simulink model "discrete_model"  (R2024b)
settings: Solver=VariableStepAuto  StartTime=0.0  StopTime=10.0  MaxStep=1e-4  RelTol=1e-3
values from neighbouring files (symbols this model uses):
  A = [0,1; 0,-10]    [conti_ss_script.m]    (also in discrete_script.m = [0,1; -3, -60]; error_space_script.m = [0,1; 0,-20]; observer_script.m = [0,1; 0,-20]; pid_script.m)
  B = [0; 120]    [conti_ss_script.m]    (also in discrete_script.m = [0; 1]; error_space_script.m = [0; 60]; observer_script.m = [0; 60]; pid_script.m)
  C = [1, 0]    [conti_ss_script.m]    (also in discrete_script.m = [90, 0]; error_space_script.m = [1,0]; observer_script.m = [1,0]; pid_script.m)
  D = 0    [conti_ss_script.m]    (also in discrete_script.m; error_space_script.m; observer_script.m; pid_script.m)
  GamO = GamOO    [discrete_script.m]
  HO = HOO    [discrete_script.m]
  JO = JOO    [discrete_script.m]
  K = Ke(2:end)    [conti_ss_script.m]    (also in discrete_script.m = Kdd; error_space_script.m = Kz(4:5); observer_script.m)
  Nu = ff(3)    [conti_ss_script.m]    (also in discrete_script.m = Nudd; observer_script.m)
  Nx = ff(1:2)    [conti_ss_script.m]    (also in discrete_script.m = Nxdd; observer_script.m)
  PhiO = PhiOO    [discrete_script.m]
  Ts = 1e-3    (= 0.001)    [discrete_script.m]
settings Model: Creator=pries  LastModifiedBy=pries

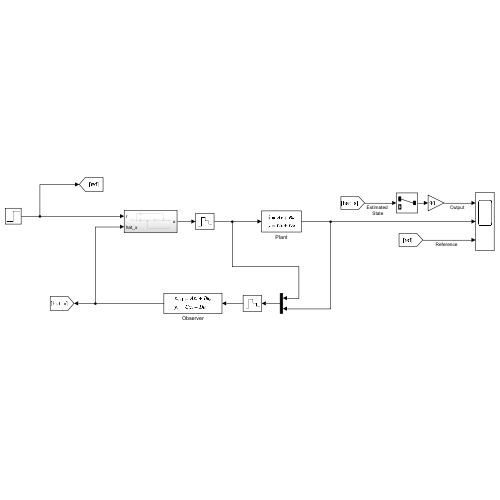
[thumbnail: Simulink's stored preview of the top-level diagram]
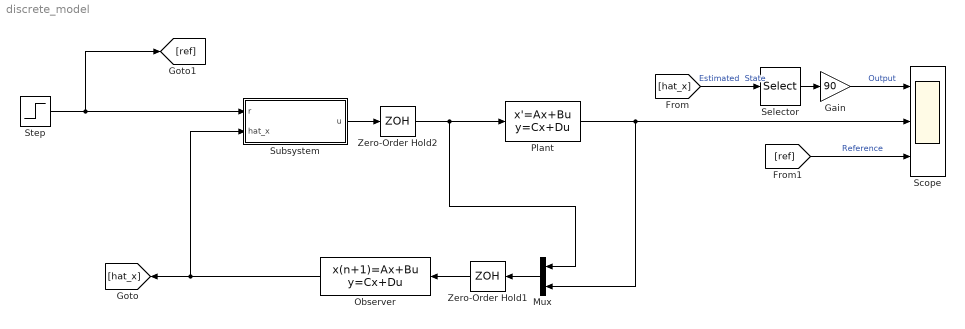
== system discrete_model ==
  Gain : Gain  Gain=90
  Mux : Mux  Inputs=2
  Observer : DiscreteStateSpace  A=PhiO  B=GamO  C=HO  D=JO  SampleTime=Ts
  Plant : StateSpace  A=A  B=B  C=C  D=D  InitialCondition=0
  Scope : Scope  NumInputPorts=3
  Selector : Selector  InputPortWidth=2  IndexOptions=Index vector (dialog)  Indices=[1]  OutputSizes=1
  Step : Step  SampleTime=0
  Subsystem : Subsystem
  Zero-Order Hold1 : ZeroOrderHold  SampleTime=-1
  Zero-Order Hold2 : ZeroOrderHold  SampleTime=-1
  wires:
  Subsystem/1(u) -> Zero-Order Hold2/1
  Mux/1 -> Zero-Order Hold1/1
  Observer/1 -> [hat_x], Subsystem/2(hat_x)
  Zero-Order Hold1/1 -> Observer/1
  Zero-Order Hold2/1 -> Mux/1, Plant/1
  Step/1 -> [ref], Subsystem/1(r)
  [ref] -> Scope/3  "Reference"
  [hat_x] -> Selector/1  "Estimated  State"
  Plant/1 -> Scope/2, Mux/2
  Selector/1 -> Gain/1
  Gain/1 -> Scope/1  "Output"

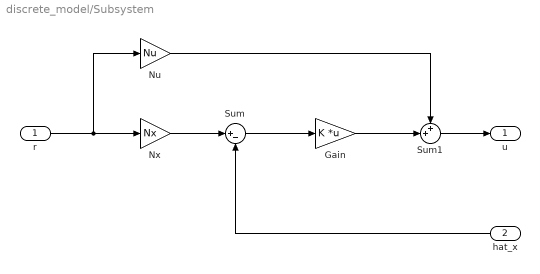
== system discrete_model/Subsystem ==
  r : Inport
  hat_x : Inport  Port=2
  Gain : Gain  Gain=K  Multiplication=Matrix(K*u)
  Nu : Gain  Gain=Nu
  Nx : Gain  Gain=Nx
  Sum : Sum  Inputs=|+-
  Sum1 : Sum  Inputs=++|
  u : Outport
  wires:
  r/1 -> Nu/1, Nx/1
  Nx/1 -> Sum/1
  Sum/1 -> Gain/1
  Sum1/1 -> u/1
  Gain/1 -> Sum1/2
  Nu/1 -> Sum1/1
  hat_x/1 -> Sum/2
